simulink model "MdEnAndBsyChk_Caller"  (R2018b)
settings: Solver=FixedStepDiscrete  StartTime=0.0  StopTime=10.0  RelTol=1e-3
undefined symbols (not defined in the file or in its folder): MdBsyClear4s_Cal, MdBsyClear6s7s_Cal, MdEnChk_Cal, MdEnClear_Cal
settings Model: Creator=sn2xws  LastModifiedBy=sn55gm
settings DataIOCC: SaveFormat=StructureWithTime
settings OptimizationCC: DefaultParameterBehavior=Inlined  EnhancedBackFolding=on  PassReuseOutputArgsAs=Individual arguments  ZeroExternalMemoryAtStartup=off  ZeroInternalMemoryAtStartup=off  OptimizeBlockOrder=speed  DifferentSizesBufferReuse=on  OptimizationCustomize=off
settings DebuggingCC: ParameterTunabilityLossMsg=error
settings SFSimCC: MATLABDynamicMemAlloc=off
settings RTWCC: SystemTargetFile=autosar.tlc  GenCodeOnly=on  TemplateMakefile=ert_default_tmf  Description=AUTOSAR  GenerateReport=on  IncludeHyperlinkInReport=on  LaunchReport=on  GenerateTraceInfo=on  GenerateTraceReport=on  GenerateTraceReportSl=on  GenerateTraceReportSf=on  GenerateTraceReportEml=on  GenerateCodeMetricsReport=on
settings CodeAppCC: ForceParamTrailComments=on  IgnoreCustomStorageClasses=off  OperatorAnnotations=on  SimulinkDataObjDesc=on  SFDataObjDesc=on  InsertBlockDesc=on
settings STFCustomTargetCC: TargetLangStandard=C99 (ISO)  MultiwordLength=256  ParMdlRefBuildCompliant=on  CompOptLevelCompliant=on  IncludeMdlTerminateFcn=off  CombineOutputUpdateFcns=on  SuppressErrorStatus=on  ERTCustomFileBanners=on  SupportNonFinite=off  SupportComplex=off  SupportContinuousTime=off  SupportNonInlinedSFcns=off  RemoveResetFunc=on  MATLABClassNameForMDSCustomization=Simulink.SoftwareTarget.ERTCustomization  AutosarCompliant=on  UseToolchainInfoCompliant=on  LookupTableObjectStructAxisOrder=2,1,3,4,...  LUTObjectStructOrderEvenSpacing=Size,Table,Breakpoints  SystemTargetFile=autosar.tlc
settings ERTTargetCC: TargetLangStandard=C99 (ISO)  ConcurrentExecutionCompliant=off  IncludeMdlTerminateFcn=off  SuppressErrorStatus=on  SupportNonFinite=off  SupportComplex=off  ModelStepFunctionPrototypeControlCompliant=off  CPPClassGenCompliant=off  AutosarCompliant=on  LookupTableObjectStructAxisOrder=2,1,3,4,...  LUTObjectStructOrderEvenSpacing=Size,Table,Breakpoints  InlinedParameterPlacement=NonHierarchical  ERTCustomFileTemplate=example_file_process.tlc  ERTFilePackagingFormat=Compact

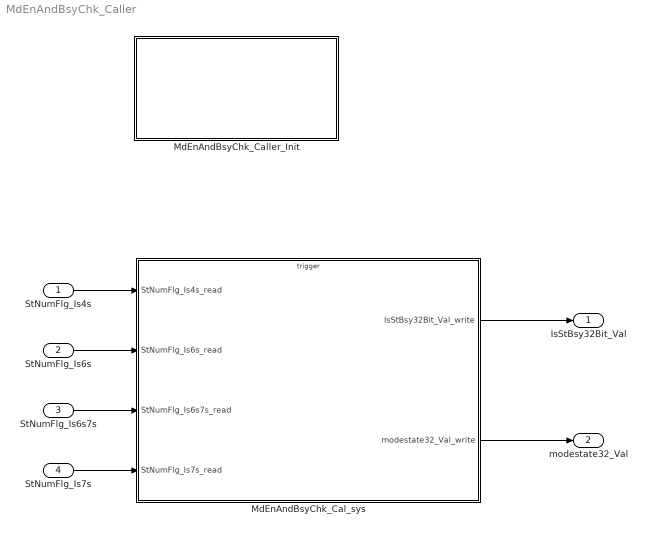
== system MdEnAndBsyChk_Caller ==
  StNumFlg_Is4s : Inport  OutDataTypeStr=boolean  PortDimensions=1
  StNumFlg_Is6s : Inport  Port=2  OutDataTypeStr=boolean  PortDimensions=1
  StNumFlg_Is6s7s : Inport  Port=3  OutDataTypeStr=boolean  PortDimensions=1
  StNumFlg_Is7s : Inport  Port=4  OutDataTypeStr=boolean  PortDimensions=1
  MdEnAndBsyChk_Cal_sys : Subsystem
  MdEnAndBsyChk_Caller_Init : Subsystem
  IsStBsy32Bit_Val : Outport  OutDataTypeStr=uint32  PortDimensions=1
  modestate32_Val : Outport  Port=2  OutDataTypeStr=uint32  PortDimensions=1
  wires:
  StNumFlg_Is4s/1 -> MdEnAndBsyChk_Cal_sys/1(StNumFlg_Is4s_read)
  StNumFlg_Is6s/1 -> MdEnAndBsyChk_Cal_sys/2(StNumFlg_Is6s_read)
  StNumFlg_Is6s7s/1 -> MdEnAndBsyChk_Cal_sys/3(StNumFlg_Is6s7s_read)
  StNumFlg_Is7s/1 -> MdEnAndBsyChk_Cal_sys/4(StNumFlg_Is7s_read)
  MdEnAndBsyChk_Cal_sys/1(IsStBsy32Bit_Val_write) -> IsStBsy32Bit_Val/1
  MdEnAndBsyChk_Cal_sys/2(modestate32_Val_write) -> modestate32_Val/1

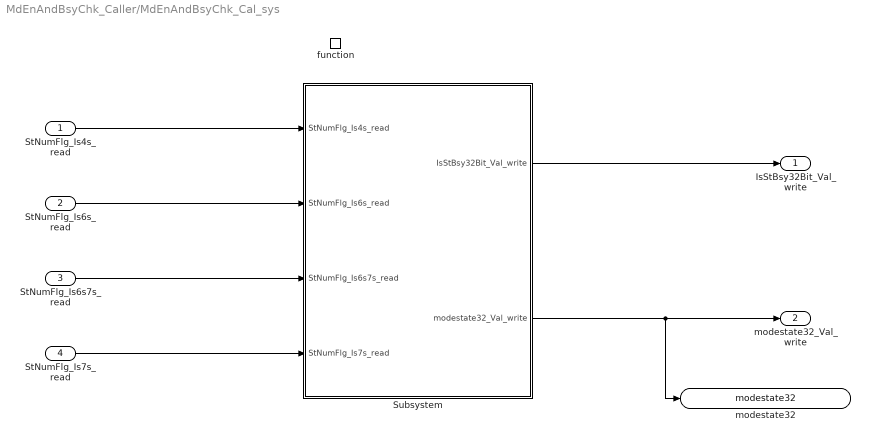
== system MdEnAndBsyChk_Caller/MdEnAndBsyChk_Cal_sys ==
  StNumFlg_Is4s_read : Inport
  StNumFlg_Is6s_read : Inport  Port=2
  StNumFlg_Is6s7s_read : Inport  Port=3
  StNumFlg_Is7s_read : Inport  Port=4
  function : TriggerPort  TriggerType=function-call  IsSimulinkFunction=on  FunctionName=MdEnAndBsyChk_Cal  VariantControl=(inherit)
  Subsystem : Subsystem
  modestate32 : ArgOut  OutDataTypeStr=uint32  ArgumentName=modestate32
  IsStBsy32Bit_Val_write : Outport
  modestate32_Val_write : Outport  Port=2  InitialOutput=0
  wires:
  StNumFlg_Is4s_read/1 -> Subsystem/1(StNumFlg_Is4s_read)
  StNumFlg_Is6s_read/1 -> Subsystem/2(StNumFlg_Is6s_read)
  StNumFlg_Is6s7s_read/1 -> Subsystem/3(StNumFlg_Is6s7s_read)
  StNumFlg_Is7s_read/1 -> Subsystem/4(StNumFlg_Is7s_read)
  Subsystem/1(IsStBsy32Bit_Val_write) -> IsStBsy32Bit_Val_write/1
  Subsystem/2(modestate32_Val_write) -> modestate32_Val_write/1, modestate32/1

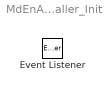
== system MdEnAndBsyChk_Caller/MdEnAndBsyChk_Caller_Init ==
  Event Listener : EventListener  EventName=reset

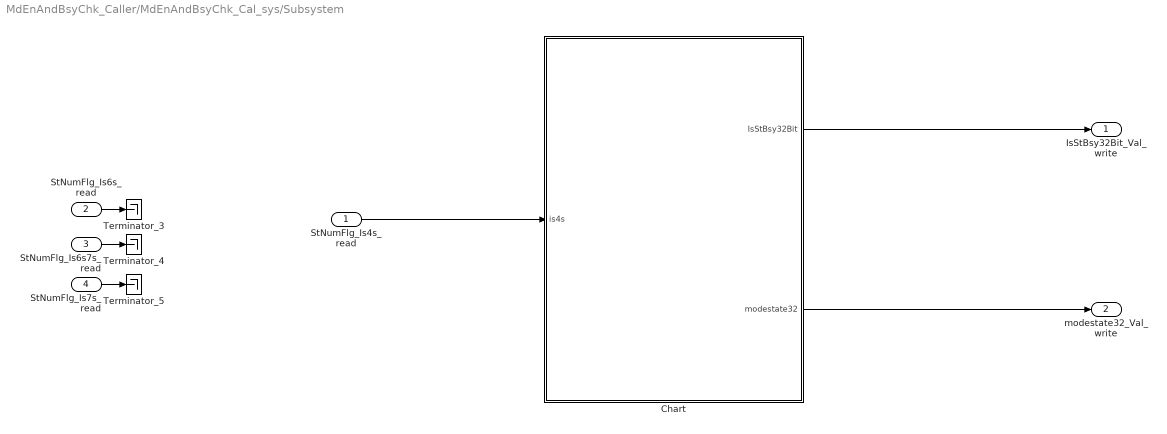
== system MdEnAndBsyChk_Caller/MdEnAndBsyChk_Cal_sys/Subsystem ==
  StNumFlg_Is4s_read : Inport
  StNumFlg_Is6s_read : Inport  Port=2
  StNumFlg_Is6s7s_read : Inport  Port=3
  StNumFlg_Is7s_read : Inport  Port=4
  Chart : Stateflow chart  TreatAsAtomicUnit=on
  Terminator_3 : Terminator
  Terminator_4 : Terminator
  Terminator_5 : Terminator
  IsStBsy32Bit_Val_write : Outport
      settings: EnsureOutportIsVirtual=on
  modestate32_Val_write : Outport  Port=2
      settings: EnsureOutportIsVirtual=on
  wires:
  StNumFlg_Is4s_read/1 -> Chart/1(is4s)
  StNumFlg_Is6s_read/1 -> Terminator_3/1
  StNumFlg_Is7s_read/1 -> Terminator_5/1
  StNumFlg_Is6s7s_read/1 -> Terminator_4/1
  Chart/1(IsStBsy32Bit) -> IsStBsy32Bit_Val_write/1
  Chart/2(modestate32) -> modestate32_Val_write/1

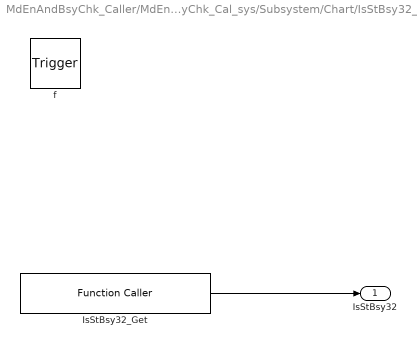
== system MdEnAndBsyChk_Caller/MdEnAndBsyChk_Cal_sys/Subsystem/Chart/IsStBsy32_Get ==
  f : TriggerPort  TriggerType=function-call  VariantControl=(inherit)
      settings: CopyFcn=Stateflow.SLINSF.SimulinkMan.removeBlockPreDeleteFcn  PreDeleteFcn=Stateflow.SLINSF.SimulinkMan.unsafePredeleteFcn
  IsStBsy32_Get : FunctionCaller  FunctionPrototype=IsStBsy32Bit = IsStBsy32_Get()  OutputArgumentSpecifications=uint32(1)
  IsStBsy32 : Outport
  wires:
  IsStBsy32_Get/1 -> IsStBsy32/1

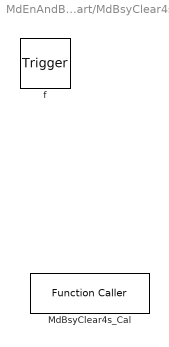
== system MdEnAndBsyChk_Caller/MdEnAndBsyChk_Cal_sys/Subsystem/Chart/MdBsyClear4s ==
  f : TriggerPort  TriggerType=function-call  VariantControl=(inherit)
      settings: CopyFcn=Stateflow.SLINSF.SimulinkMan.removeBlockPreDeleteFcn  PreDeleteFcn=Stateflow.SLINSF.SimulinkMan.unsafePredeleteFcn
  MdBsyClear4s_Cal : FunctionCaller  FunctionPrototype=MdBsyClear4s_Cal()

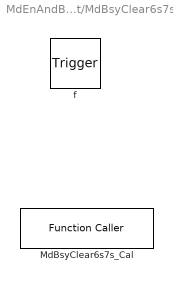
== system MdEnAndBsyChk_Caller/MdEnAndBsyChk_Cal_sys/Subsystem/Chart/MdBsyClear6s7s ==
  f : TriggerPort  TriggerType=function-call  VariantControl=(inherit)
      settings: CopyFcn=Stateflow.SLINSF.SimulinkMan.removeBlockPreDeleteFcn  PreDeleteFcn=Stateflow.SLINSF.SimulinkMan.unsafePredeleteFcn
  MdBsyClear6s7s_Cal : FunctionCaller  FunctionPrototype=MdBsyClear6s7s_Cal()

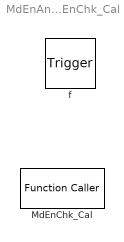
== system MdEnAndBsyChk_Caller/MdEnAndBsyChk_Cal_sys/Subsystem/Chart/MdEnChk_Cal ==
  f : TriggerPort  TriggerType=function-call  VariantControl=(inherit)
      settings: CopyFcn=Stateflow.SLINSF.SimulinkMan.removeBlockPreDeleteFcn  PreDeleteFcn=Stateflow.SLINSF.SimulinkMan.unsafePredeleteFcn
  MdEnChk_Cal : FunctionCaller  Description=|  FunctionPrototype=MdEnChk_Cal()
      | StNun: 
      | 0 :4s
      | 1:6s
      | 2:7s
      | 3:4sp

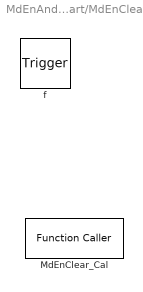
== system MdEnAndBsyChk_Caller/MdEnAndBsyChk_Cal_sys/Subsystem/Chart/MdEnClear ==
  f : TriggerPort  TriggerType=function-call  VariantControl=(inherit)
      settings: CopyFcn=Stateflow.SLINSF.SimulinkMan.removeBlockPreDeleteFcn  PreDeleteFcn=Stateflow.SLINSF.SimulinkMan.unsafePredeleteFcn
  MdEnClear_Cal : FunctionCaller  FunctionPrototype=MdEnClear_Cal()

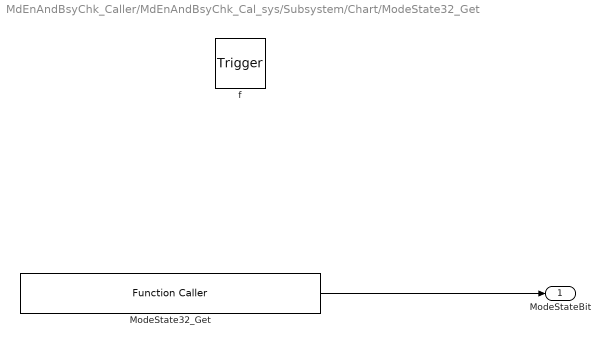
== system MdEnAndBsyChk_Caller/MdEnAndBsyChk_Cal_sys/Subsystem/Chart/ModeState32_Get ==
  f : TriggerPort  TriggerType=function-call  VariantControl=(inherit)
      settings: CopyFcn=Stateflow.SLINSF.SimulinkMan.removeBlockPreDeleteFcn  PreDeleteFcn=Stateflow.SLINSF.SimulinkMan.unsafePredeleteFcn
  ModeState32_Get : FunctionCaller  FunctionPrototype=MdEn32 = ModeState32_Get()  OutputArgumentSpecifications=uint32(1)
  ModeStateBit : Outport
  wires:
  ModeState32_Get/1 -> ModeStateBit/1

== stateflow chart MdEnAndBsyChk_Caller/MdEnAndBsyChk_Cal_sys/Subsystem/Chart ==
  state MdEnClear [function]
  state MdBsyClear4s [function]
  state MdEnChk_Cal [function]
  state MdBsyClear6s7s [function]
  state IsStBsy32 =IsStBsy32_Get [function]
  state ModeStateBit =ModeState32_Get [function]
  (default) -> (junction 1)
  (junction 1) -> (junction 7) : {
      | MdEnClear();
      | }
  (junction 7) -> (junction 9) [order 1] : [is4s]
  (junction 7) -> (junction 19) [order 2] : {
      | MdBsyClear6s7s();
      | MdEnChk_Cal();
      | }
  (junction 9) -> (junction 16) : {
      | MdBsyClear4s();
      | MdEnChk_Cal();
      | }
  (junction 16) -> (junction 19)
  (junction 19) -> (junction 22) : {
      | IsStBsy32Bit = IsStBsy32_Get();
      | modestate32 =ModeState32_Get();
      | }
  data: IsStBsy32 function_output; ModeStateBit function_output; is4s input; IsStBsy32Bit output; modestate32 output
